simulink model "block_sensorless_startup_SMO_R2018a_sim_2020817"  (R2018a)
settings: Solver=ode1  StartTime=0.0  StopTime=1  FixedStep=1e-6  RelTol=1e-3  EnableMultiTasking=on
PreLoadFcn:
  | Psif= 0.003234246776455;  %magnet
  | Lq0 = 118e-6/2;  %inductance of q axis
  | Ld0 = 52.6e-6/2;   %inductance of d axis
  | R   =  43.73*0.5e-3;
  | 
  | Pn=4;       %poles pairs number
  | pi=3.1415926;
  | 
  | J=1.658254e-5*5;
  | Vdc=18;
undefined symbols (not defined in the file): DiscIntNeverNeededParam
libraries: powerlib x9, simulink x1
CloseFcn:
  | rtwprivate ssgencode ModelCloseRequest BLDC_baby_stroll_new_start
settings Model: DSRTSU_INTERNAL_RTI_VER=390  DSRTSU_INTERNAL_RTI_TYPE=rti1005  Creator=Engineer  LastModifiedBy=JinHua Luo
settings DataIOCC: LimitDataPoints=on  SaveFormat=Array  SignalLoggingSaveFormat=ModelDataLogs
settings OptimizationCC: BlockReduction=off  ConditionallyExecuteInputs=off  OptimizeBlockIOStorage=off  BufferReuse=off  GlobalBufferReuse=off  ExpressionFolding=off  EnableMemcpy=off  ExpressionDepthLimit=2147483647  LocalBlockOutputs=off  InitFltsAndDblsToZero=on  LifeSpan=inf  SimCompilerOptimization=on  OptimizeDataStoreBuffers=off  BusAssignmentInplaceUpdate=off
settings DebuggingCC: UnderspecifiedInitializationDetection=Classic  MergeDetectMultiDrivingBlocksExec=none  SolverPrmCheckMsg=warning  FcnCallInpInsideContextMsg=warning  StateNameClashWarn=warning  SFUnexpectedBacktrackingDiag=warning  SFNoUnconditionalDefaultTransitionDiag=warning  SFExecutionAtInitializationDiag=none
settings HardwareCC: ProdBitPerPointer=32  ProdBitPerSizeT=32  ProdBitPerPtrDiffT=32  ProdLargestAtomicFloat=None  ProdEndianess=BigEndian  ProdWordSize=32  ProdHWDeviceType=Generic->Custom  TargetIntDivRoundTo=Zero  TargetEndianess=BigEndian  TargetHWDeviceType=Generic->Custom
settings ModelReferenceCC: PropagateSignalLabelsOutOfModel=off
settings RTWCC: SystemTargetFile=rti1005.tlc  MakeCommand=make_rti  TemplateMakefile=rti1005.tmf  Description=dSPACE DS1005 Hardware Platform
settings CodeAppCC: StateflowObjectComments=on
settings STFCustomTargetCC: ParMdlRefBuildCompliant=on  GeneratePreprocessorConditionals=Disable all  CPPClassGenCompliant=on  SystemTargetFile=rti1005.tlc
settings GRTTargetCC: TargetLangStandard=C89/C90 (ANSI)  CompOptLevelCompliant=off  ConcurrentExecutionCompliant=off  GeneratePreprocessorConditionals=Disable all  CombineOutputUpdateFcns=off  MatFileLogging=off  GRTInterface=on  UseToolchainInfoCompliant=off  ExtModeMexFile=noextcomm
settings ConfigComp: CovMetricSettings=dw  CovHtmlReporting=on  CovSaveCumulativeToWorkspaceVar=on  CovSaveSingleToWorkspaceVar=on  CovExternalEMLEnable=off
settings SimscapeCC: SimscapeNormalizeSystem=off

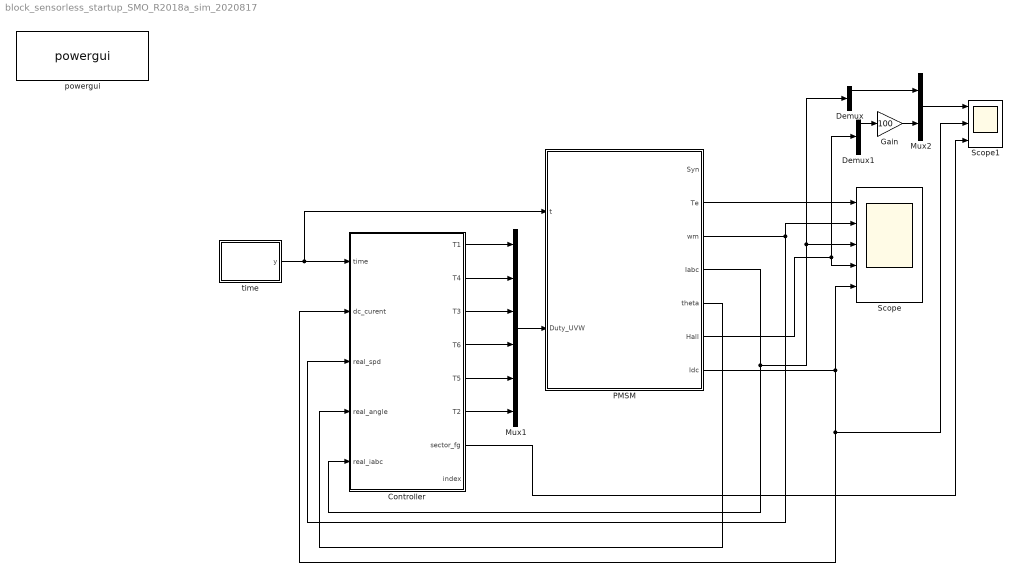
== system block_sensorless_startup_SMO_R2018a_sim_2020817 ==
  Controller : Subsystem
  Demux : Demux  Outputs=3
  Demux1 : Demux  Outputs=3
  Gain : Gain  Gain=100
  Mux1 : Mux  Inputs=6
  Mux2 : Mux  Inputs=2
  PMSM : Subsystem
  Scope : Scope  NumInputPorts=5
  Scope1 : Scope  NumInputPorts=3
  powergui : powerlib/powergui  Priority=2  SimulationMode=Discrete  SampleTime=1e-6  frequency=60  Iterations=50  frequencyindice=0  Pbase=100e6  ErrMax=1e-4  UnitsV=kV  UnitsW=MW  buscounter=0  FunctionMessages=off  echomessages=off  EnableUseOfTLC=off  CurrentSourceSwitches=off  DisableSnubberDevices=off  DisableRonSwitches=off  DisableVfSwitches=off  DisplayEquations=off  SolverType=Tustin/Backward Euler (TBE)  Interpol=off  ExternalGateDelay=off  methode=off  Ts=0  x0status=blocks  SPID=off  SwTol=0  HookPort=off  RestoreLinks=warning  ResistiveCurrentMeasurement=off  Frange=[0:2:500]  Ylog=off  Xlog=on  ShowGrid=off  save=off  variable=ZData  structure=0  ZoomFFT=on  StartTime=0.0  cycles=1  DisplayStyle=1  fundamental=60  FreqAxis=off  MaxFrequency=1000  frequencyindicesteady=1  RmsSteady=1  display=off
  time : MATLAB Function  TreatAsAtomicUnit=on
  wires:
  time/1(y) -> PMSM/1(t), Controller/1(time)
  Controller/1(T1) -> Mux1/1
  Controller/2(T4) -> Mux1/2
  Controller/3(T3) -> Mux1/3
  Controller/4(T6) -> Mux1/4
  Controller/5(T5) -> Mux1/5
  Controller/6(T2) -> Mux1/6
  Mux1/1 -> PMSM/2(Duty_UVW)
  PMSM/7(Idc) -> Scope/5, Controller/2(dc_curent), Scope1/2
  PMSM/2(Te) -> Scope/1
  PMSM/3(wm) -> Scope/2, Controller/3(real_spd)
  PMSM/4(Iabc) -> Controller/5(real_iabc), Demux/1, Scope/3
  PMSM/6(Hall) -> Demux1/1, Scope/4
  Demux/1 -> Mux2/1
  Demux1/1 -> Gain/1
  Mux2/1 -> Scope1/1
  Gain/1 -> Mux2/2
  Controller/7(sector_fg) -> Scope1/3
  PMSM/5(theta) -> Controller/4(real_angle)

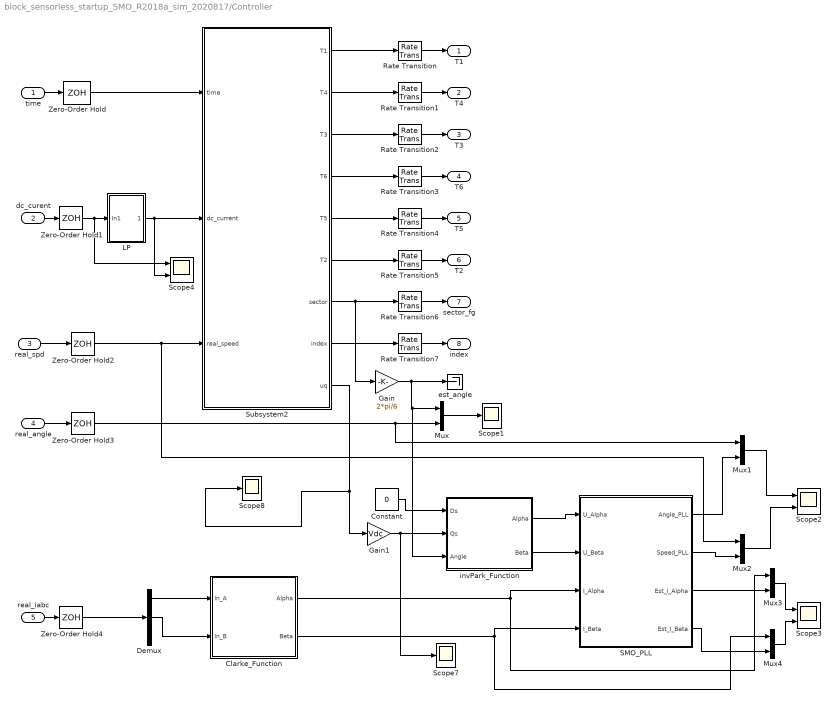
== system block_sensorless_startup_SMO_R2018a_sim_2020817/Controller ==
  time : Inport
  dc_curent : Inport  Port=2
  real_spd : Inport  Port=3
  real_angle : Inport  Port=4
  real_iabc : Inport  Port=5
  Clarke_Function : MATLAB Function  TreatAsAtomicUnit=on
  Constant : Constant  Value=0
  Demux : Demux  Outputs=3
  Gain : Gain  Gain=2*pi/6
  Gain1 : Gain  Gain=Vdc
  LP : Subsystem
  Mux{,1..4} (5 alike) : Mux  Inputs=2
  Rate Transition{,1..7} (8 alike) : RateTransition
  SMO_PLL : Subsystem
  Scope1 : Scope
  Scope2 : Scope  NumInputPorts=2
  Scope3 : Scope  NumInputPorts=2
  Scope4 : Scope  NumInputPorts=2
  Scope7 : Scope
  Scope8 : Scope
  Subsystem2 : Subsystem
  Zero-Order Hold{,1..4} (5 alike) : ZeroOrderHold  SampleTime=5e-5
  est_angle : Terminator
  invPark_Function : MATLAB Function  TreatAsAtomicUnit=on
  T1 : Outport
  T4 : Outport  Port=2
  T3 : Outport  Port=3
  T6 : Outport  Port=4
  T5 : Outport  Port=5
  T2 : Outport  Port=6
  sector_fg : Outport  Port=7
  index : Outport  Port=8
  wires:
  Subsystem2/1(T1) -> Rate Transition/1
  Subsystem2/2(T4) -> Rate Transition1/1
  Subsystem2/3(T3) -> Rate Transition2/1
  Subsystem2/4(T6) -> Rate Transition3/1
  Subsystem2/5(T5) -> Rate Transition4/1
  Subsystem2/6(T2) -> Rate Transition5/1
  time/1 -> Zero-Order Hold/1
  dc_curent/1 -> Zero-Order Hold1/1
  LP/1(Out1) -> Scope4/2, Subsystem2/2(dc_current)
  Zero-Order Hold/1 -> Subsystem2/1(time)
  Zero-Order Hold1/1 -> LP/1(In1), Scope4/1
  Rate Transition/1 -> T1/1
  Rate Transition1/1 -> T4/1
  Rate Transition2/1 -> T3/1
  Rate Transition3/1 -> T6/1
  Rate Transition4/1 -> T5/1
  Rate Transition5/1 -> T2/1
  Rate Transition6/1 -> sector_fg/1
  Rate Transition7/1 -> index/1
  Subsystem2/8(index) -> Rate Transition7/1
  real_spd/1 -> Zero-Order Hold2/1
  Zero-Order Hold2/1 -> Mux2/1, Subsystem2/3(real_speed)
  real_angle/1 -> Zero-Order Hold3/1
  real_iabc/1 -> Zero-Order Hold4/1
  Subsystem2/7(sector) -> Gain/1, Rate Transition6/1
  Gain/1 -> est_angle/1, invPark_Function/3(Angle), Mux/1
  Mux/1 -> Scope1/1
  Zero-Order Hold3/1 -> Mux1/1, Mux/2
  Demux/1 -> Clarke_Function/1(In_A)
  Demux/2 -> Clarke_Function/2(In_B)
  Clarke_Function/1(Alpha) -> SMO_PLL/3(I_Alpha), Mux3/1
  Clarke_Function/2(Beta) -> SMO_PLL/4(I_Beta), Mux4/1
  Subsystem2/9(uq) -> Scope8/1, Gain1/1
  invPark_Function/1(Alpha) -> SMO_PLL/1(U_Alpha)
  invPark_Function/2(Beta) -> SMO_PLL/2(U_Beta)
  Constant/1 -> invPark_Function/1(Ds)
  SMO_PLL/1(Angle_PLL) -> Mux1/2
  Mux1/1 -> Scope2/1
  SMO_PLL/2(Speed_PLL) -> Mux2/2
  Mux2/1 -> Scope2/2
  SMO_PLL/3(Est_I_Alpha) -> Mux3/2
  SMO_PLL/4(Est_I_Beta) -> Mux4/2
  Mux3/1 -> Scope3/1
  Mux4/1 -> Scope3/2
  Gain1/1 -> Scope7/1, invPark_Function/2(Qs)
  Zero-Order Hold4/1 -> Demux/1

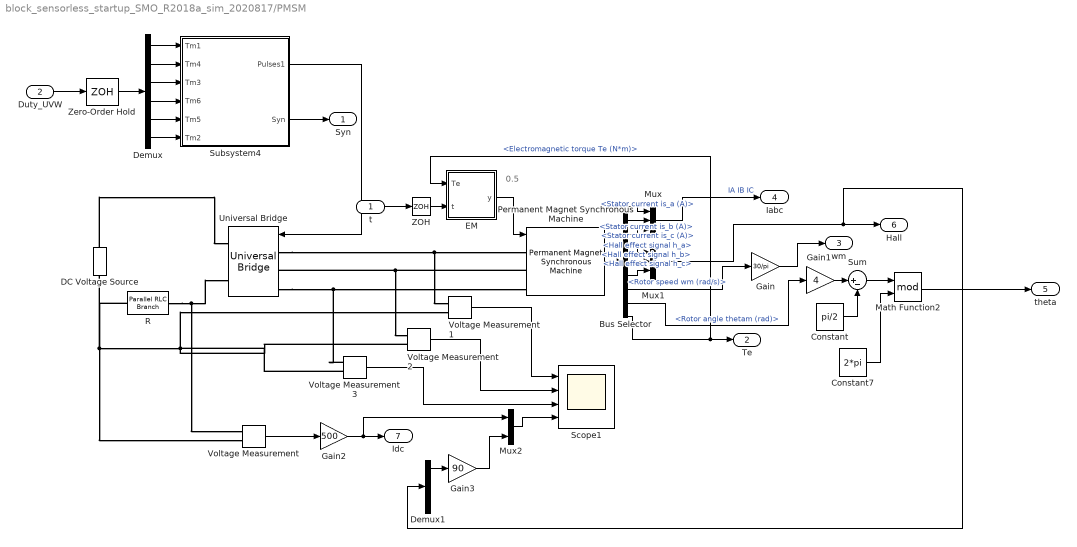
== system block_sensorless_startup_SMO_R2018a_sim_2020817/PMSM ==
  note: 0.5
  t : Inport
  Duty_UVW : Inport  Port=2  OutDataTypeStr=double
  Bus Selector : BusSelector  OutputSignals=Stator current is_a (A),Stator current is_b (A),Stator current is_c (A),Hall effect signal h_a,Hall effect signal h_b,Hall effect signal h_c,Rotor speed wm (rad/s),Rotor angle thetam (rad),Electromagnetic torque Te (N*m)
  Constant : Constant  Value=pi/2
  Constant7 : Constant  Value=2*pi
  DC Voltage Source : powerlib/Electrical Sources/DC Voltage Source  Amplitude=Vdc  Measurements=None
  Demux : Demux  Outputs=6
  Demux1 : Demux  Outputs=3
  EM : MATLAB Function  TreatAsAtomicUnit=on
  Gain : Gain  Gain=30/pi
  Gain1 : Gain  Gain=4
  Gain2 : Gain  Gain=500
  Gain3 : Gain  Gain=90
  Math Function2 : Math  Operator=mod  SaturateOnIntegerOverflow=on
  Mux : Mux  Inputs=3
  Mux1 : Mux  Inputs=3
  Mux2 : Mux  Inputs=2
  Permanent Magnet Synchronous Machine : powerlib/Machines/Permanent Magnet Synchronous Machine  NbPhases=3  FluxDistribution=Sinusoidal  RotorType=Salient-pole  MechanicalLoad=Torque Tm  PresetModel=No  ShowDetailedParameters=on  MeasurementBus=off  Resistance=R  Inductance=8.5e-3  dqInductances=[Ld0,Lq0]  La=0.000395  MachineConstant=Flux linkage established by magnets (V.s)  Flux=Psif  VoltageCst=2.3465  TorqueCst=0.019405  Flat=120  Mechanical=[J 100e-5 4]  PolePairs=4  InitialConditions=[0,0, 0,0]  InitialConditions5ph=[0 0 0 0 0 0]  TsPowergui=0  TsBlock=-1  RefAngle=90 degrees behind phase A axis (modified Park)
      settings: SourceProductName=Simscape Power Systems
  R : powerlib/Elements/Parallel RLC Branch  LConnTagsString=a  RConnTagsString=__new0  BranchType=R  Resistance=0.002  Inductance=1e-3  SetiL0=off  InitialCurrent=0  Capacitance=1e-6  Setx0=off  InitialVoltage=0  Measurements=None
  Scope1 : Scope  NumInputPorts=4
  Subsystem4 : Subsystem
  Sum : Sum  Inputs=|+-
  Universal Bridge : powerlib/Power Electronics/Universal Bridge  Arms=3  SnubberResistance=100  SnubberCapacitance=1e-5  Device=MOSFET / Diodes  Ron=3e-3  Lon=0  ForwardVoltages="[  0  0  ]"  ForwardVoltage=0  GTOparameters=[ 10e-6 , 20e-6 ]  IGBTparameters=[ 1e-6 , 2e-6 ]  Measurements=None  Measurements_2=None  converterType=Rectifier
  Voltage Measurement{,1..3} (4 alike) : powerlib/Measurements/Voltage Measurement  PhasorSimulation=off  OutputType=Complex  PSBequivalent=0
  ZOH : ZeroOrderHold  SampleTime=1e-6
  Zero-Order Hold : ZeroOrderHold  SampleTime=1e-6
  Syn : Outport
  Te : Outport  Port=2
  wm : Outport  Port=3
  Iabc : Outport  Port=4
  theta : Outport  Port=5
  Hall : Outport  Port=6
  Idc : Outport  Port=7
  wires:
  Permanent Magnet Synchronous Machine/1 -> Bus Selector/1
  Mux/1 -> Iabc/1  "IA IB IC"
  Bus Selector/7 -> Gain/1  "<Rotor speed wm (rad/s)>"
  Bus Selector/9 -> EM/1(Te), Te/1  "<Electromagnetic torque Te (N*m)>"
  Subsystem4/1(Pulses1) -> Universal Bridge/1
  Duty_UVW/1 -> Zero-Order Hold/1
  Subsystem4/2(Syn) -> Syn/1
  Constant/1 -> Sum/2
  Constant7/1 -> Math Function2/2
  Bus Selector/8 -> Gain1/1  "<Rotor angle thetam (rad)>"
  Math Function2/1 -> theta/1
  Gain/1 -> wm/1
  t/1 -> ZOH/1
  Demux/6 -> Subsystem4/6(Tm2)
  Demux/5 -> Subsystem4/5(Tm5)
  Demux/4 -> Subsystem4/4(Tm6)
  Demux/3 -> Subsystem4/3(Tm3)
  Demux/2 -> Subsystem4/2(Tm4)
  Demux/1 -> Subsystem4/1(Tm1)
  Zero-Order Hold/1 -> Demux/1
  ZOH/1 -> EM/2(t)
  Voltage Measurement/1 -> Gain2/1
  Gain2/1 -> Mux2/1, Idc/1
  EM/1(y) -> Permanent Magnet Synchronous Machine/1
  Mux1/1 -> Hall/1, Demux1/1
  Voltage Measurement1/1 -> Scope1/1
  Bus Selector/3 -> Mux/3  "<Stator current is_c (A)>"
  Bus Selector/2 -> Mux/2  "<Stator current is_b (A)>"
  Bus Selector/1 -> Mux/1  "<Stator current is_a (A)>"
  Bus Selector/5 -> Mux1/2  "<Hall effect signal h_b>"
  Bus Selector/6 -> Mux1/3  "<Hall effect signal h_c>"
  Bus Selector/4 -> Mux1/1  "<Hall effect signal h_a>"
  Voltage Measurement2/1 -> Scope1/2
  Voltage Measurement3/1 -> Scope1/3
  Demux1/1 -> Gain3/1
  Gain3/1 -> Mux2/2
  Mux2/1 -> Scope1/4
  Gain1/1 -> Sum/1
  Sum/1 -> Math Function2/1
  connections:
  Universal Bridge/LConn1 -- Permanent Magnet Synchronous Machine/LConn1 -- Voltage Measurement1/LConn1
  Permanent Magnet Synchronous Machine/LConn2 -- Universal Bridge/LConn2 -- Voltage Measurement2/LConn1
  Universal Bridge/LConn3 -- Voltage Measurement3/LConn1 -- Permanent Magnet Synchronous Machine/LConn3
  DC Voltage Source/RConn1 -- Universal Bridge/RConn1
  R/RConn1 -- Universal Bridge/RConn2 -- Voltage Measurement/LConn1
  R/LConn1 -- DC Voltage Source/LConn1 -- Voltage Measurement/LConn2 -- Voltage Measurement2/LConn2 -- Voltage Measurement3/LConn2 -- Voltage Measurement1/LConn2

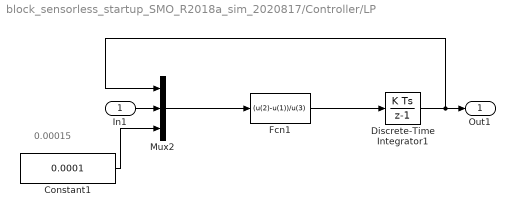
== system block_sensorless_startup_SMO_R2018a_sim_2020817/Controller/LP ==
  note: 0.00015
  In1 : Inport
  Constant1 : Constant  Value=0.0001  SampleTime=-1
  Discrete-Time Integrator1 : DiscreteIntegrator  SampleTime=-1  ICPrevOutput=DiscIntNeverNeededParam  ICPrevScaledInput=DiscIntNeverNeededParam
  Fcn1 : Fcn  Expr=(u(2)-u(1))/u(3)
  Mux2 : Mux  Inputs=3
  Out1 : Outport
  wires:
  Constant1/1 -> Mux2/3
  Mux2/1 -> Fcn1/1
  Fcn1/1 -> Discrete-Time Integrator1/1
  Discrete-Time Integrator1/1 -> Mux2/1, Out1/1
  In1/1 -> Mux2/2

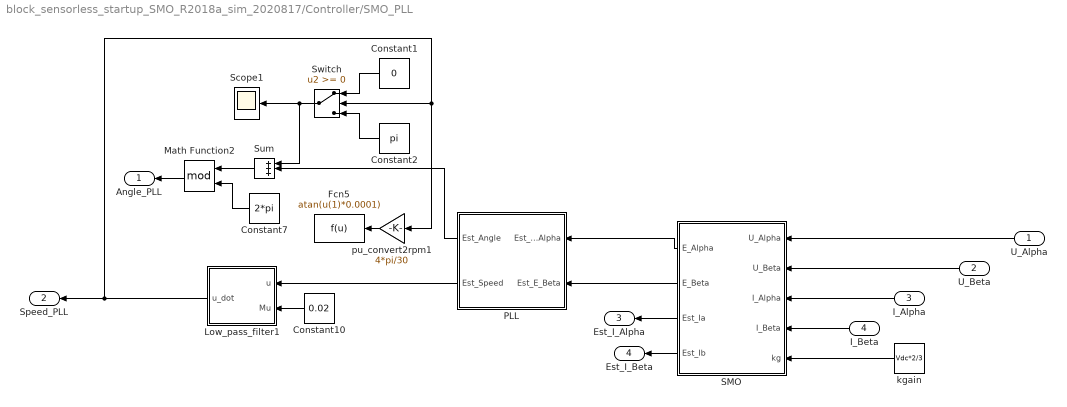
== system block_sensorless_startup_SMO_R2018a_sim_2020817/Controller/SMO_PLL ==
  U_Alpha : Inport
  U_Beta : Inport  Port=2
  I_Alpha : Inport  Port=3
  I_Beta : Inport  Port=4
  Constant1 : Constant  Value=0
  Constant10 : Constant  Value=0.02
  Constant2 : Constant  Value=pi
  Constant7 : Constant  Value=2*pi
  Fcn5 : Fcn  Expr=atan(u(1)*0.0001)
  Low_pass_filter1 : Subsystem
  Math Function2 : Math  Operator=mod  SaturateOnIntegerOverflow=on
  PLL : MATLAB Function  TreatAsAtomicUnit=on
  SMO : MATLAB Function  TreatAsAtomicUnit=on
  Scope1 : Scope
  Sum : Sum  Inputs=+++
  Switch : Switch
  kgain : Constant  Value=Vdc*2/3
  pu_convert2rpm1 : Gain  Gain=4*pi/30
  Angle_PLL : Outport
  Speed_PLL : Outport  Port=2
  Est_I_Alpha : Outport  Port=3
  Est_I_Beta : Outport  Port=4
  wires:
  Low_pass_filter1/1(u_dot) -> Speed_PLL/1, Switch/2, pu_convert2rpm1/1
  Constant10/1 -> Low_pass_filter1/2(Mu)
  I_Beta/1 -> SMO/4(I_Beta)
  I_Alpha/1 -> SMO/3(I_Alpha)
  U_Beta/1 -> SMO/2(U_Beta)
  U_Alpha/1 -> SMO/1(U_Alpha)
  Constant7/1 -> Math Function2/2
  PLL/2(Est_Speed) -> Low_pass_filter1/1(u)
  kgain/1 -> SMO/5(kg)
  Sum/1 -> Math Function2/1
  pu_convert2rpm1/1 -> Fcn5/1
  Math Function2/1 -> Angle_PLL/1
  SMO/1(E_Alpha) -> PLL/1(Est_E_Alpha)
  SMO/2(E_Beta) -> PLL/2(Est_E_Beta)
  PLL/1(Est_Angle) -> Sum/2
  Switch/1 -> Sum/1, Scope1/1
  SMO/4(Est_Ib) -> Est_I_Beta/1
  SMO/3(Est_Ia) -> Est_I_Alpha/1
  Constant2/1 -> Switch/3
  Constant1/1 -> Switch/1

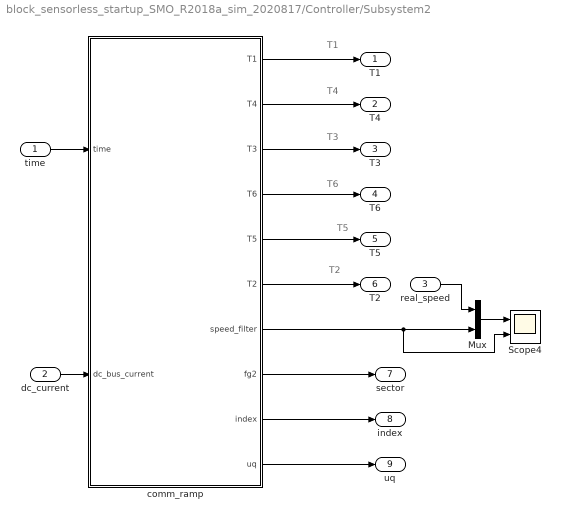
== system block_sensorless_startup_SMO_R2018a_sim_2020817/Controller/Subsystem2 ==
  note: T1
  note: T4
  note: T3
  note: T6
  note: T5
  note: T2
  time : Inport
  dc_current : Inport  Port=2
  real_speed : Inport  Port=3
  Mux : Mux  Inputs=2
  Scope4 : Scope  NumInputPorts=2
  comm_ramp : Subsystem  SystemSampleTime=4e-5
  T1 : Outport
  T4 : Outport  Port=2
  T3 : Outport  Port=3
  T6 : Outport  Port=4
  T5 : Outport  Port=5
  T2 : Outport  Port=6
  sector : Outport  Port=7
  index : Outport  Port=8
  uq : Outport  Port=9
  wires:
  time/1 -> comm_ramp/1(time)
  comm_ramp/1(T1) -> T1/1
  comm_ramp/2(T4) -> T4/1
  comm_ramp/3(T3) -> T3/1
  comm_ramp/4(T6) -> T6/1
  comm_ramp/6(T2) -> T2/1
  comm_ramp/5(T5) -> T5/1
  dc_current/1 -> comm_ramp/2(dc_bus_current)
  comm_ramp/9(index) -> index/1
  real_speed/1 -> Mux/1
  comm_ramp/7(speed_filter) -> Mux/2, Scope4/2
  Mux/1 -> Scope4/1
  comm_ramp/8(fg2) -> sector/1
  comm_ramp/10(uq) -> uq/1

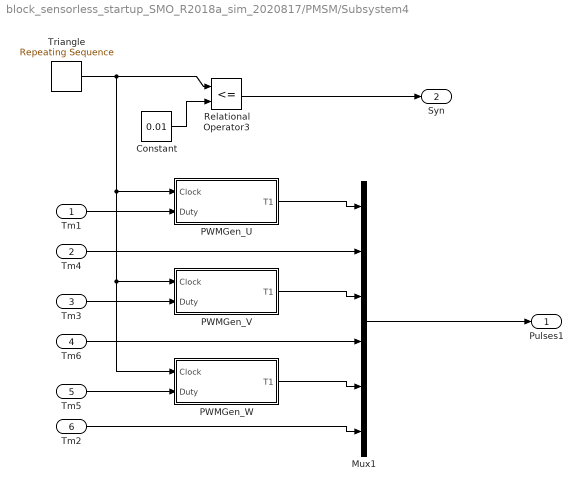
== system block_sensorless_startup_SMO_R2018a_sim_2020817/PMSM/Subsystem4 ==
  Tm1 : Inport
  Tm4 : Inport  Port=2
  Tm3 : Inport  Port=3
  Tm6 : Inport  Port=4
  Tm5 : Inport  Port=5
  Tm2 : Inport  Port=6
  Constant : Constant  Value=0.01
  Mux1 : Mux  Inputs=6
  PWMGen_U : Subsystem
  PWMGen_V : Subsystem
  PWMGen_W : Subsystem
  Relational Operator3 : RelationalOperator  Operator=<=  OutDataTypeStr=boolean  RndMeth=Nearest
  Triangle : simulink/Sources/Repeating Sequence  rep_seq_t=[0 0.000025 0.00005]  rep_seq_y=[0 1 0]
  Pulses1 : Outport
  Syn : Outport  Port=2
  wires:
  Mux1/1 -> Pulses1/1
  Tm1/1 -> PWMGen_U/2(Duty)
  Triangle/1 -> Relational Operator3/1, PWMGen_U/1(Clock), PWMGen_V/1(Clock), PWMGen_W/1(Clock)
  Relational Operator3/1 -> Syn/1
  Constant/1 -> Relational Operator3/2
  PWMGen_U/1(T1) -> Mux1/1
  Tm4/1 -> Mux1/2
  Tm2/1 -> Mux1/6
  Tm6/1 -> Mux1/4
  Tm3/1 -> PWMGen_V/2(Duty)
  Tm5/1 -> PWMGen_W/2(Duty)
  PWMGen_V/1(T1) -> Mux1/3
  PWMGen_W/1(T1) -> Mux1/5

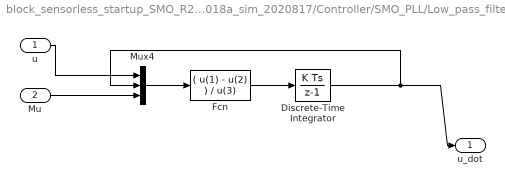
== system block_sensorless_startup_SMO_R2018a_sim_2020817/Controller/SMO_PLL/Low_pass_filter1 ==
  u : Inport
  Mu : Inport  Port=2
  Discrete-Time Integrator : DiscreteIntegrator  SampleTime=-1  RndMeth=Round  ICPrevOutput=DiscIntNeverNeededParam  ICPrevScaledInput=DiscIntNeverNeededParam
  Fcn : Fcn  Expr=( u(1) - u(2) ) / u(3)
  Mux4 : Mux  Inputs=3
  u_dot : Outport
  wires:
  Mu/1 -> Mux4/3
  u/1 -> Mux4/1
  Discrete-Time Integrator/1 -> u_dot/1, Mux4/2
  Fcn/1 -> Discrete-Time Integrator/1
  Mux4/1 -> Fcn/1

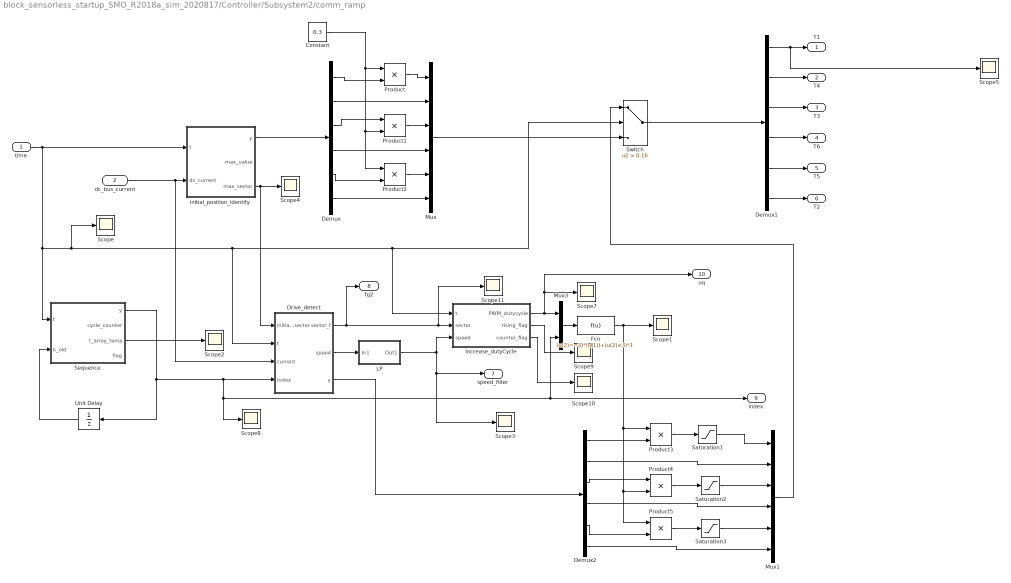
== system block_sensorless_startup_SMO_R2018a_sim_2020817/Controller/Subsystem2/comm_ramp ==
  time : Inport
  dc_bus_current : Inport  Port=2
  Constant : Constant  Value=0.3
  Demux : Demux  Outputs=6
  Demux1 : Demux  Outputs=6
  Demux2 : Demux  Outputs=6
  Drive_detect : MATLAB Function  TreatAsAtomicUnit=on
  Fcn : Fcn  Expr=(u(2)==3)*(u(1))+(u(2)<3)*1
  LP : Subsystem
  Mux : Mux  Inputs=6
  Mux1 : Mux  Inputs=6
  Mux3 : Mux  Inputs=2
  Product{,1..5} (6 alike) : Product  RndMeth=Zero
  Saturation1 : Saturate  UpperLimit=1  LowerLimit=0
  Saturation2 : Saturate  UpperLimit=1  LowerLimit=0
  Saturation3 : Saturate  UpperLimit=1  LowerLimit=0
  Scope{,1..5,7..11} (11 alike) : Scope
  Sequence : MATLAB Function  TreatAsAtomicUnit=on
  Switch : Switch  Criteria=u2 > Threshold  Threshold=0.16  OutDataTypeStr=double
  Unit Delay : UnitDelay  SampleTime=-1
  increase_dutyCycle : MATLAB Function  TreatAsAtomicUnit=on
  initial_position_identify : MATLAB Function  TreatAsAtomicUnit=on
  T1 : Outport
  T4 : Outport  Port=2
  T3 : Outport  Port=3
  T6 : Outport  Port=4
  T5 : Outport  Port=5
  T2 : Outport  Port=6
  speed_filter : Outport  Port=7
  fg2 : Outport  Port=8
  index : Outport  Port=9
  uq : Outport  Port=10
  wires:
  Demux/1 -> Product/2
  Demux/3 -> Product1/1
  Demux/5 -> Product2/2
  Constant/1 -> Product2/1, Product1/2, Product/1
  Demux1/1 -> Scope5/1, T1/1
  Demux1/2 -> T4/1
  Demux1/3 -> T3/1
  Demux1/4 -> T6/1
  Demux1/5 -> T5/1
  Demux1/6 -> T2/1
  Product/1 -> Mux/1
  Demux/2 -> Mux/2
  Product1/1 -> Mux/3
  Demux/4 -> Mux/4
  Product2/1 -> Mux/5
  Demux/6 -> Mux/6
  Mux/1 -> Switch/3
  Demux2/5 -> Product5/2
  dc_bus_current/1 -> Drive_detect/3(current), initial_position_identify/2(dc_current)
  initial_position_identify/1(y) -> Demux/1
  Demux2/3 -> Product4/1
  Product3/1 -> Saturation1/1
  Demux2/2 -> Mux1/2
  Product4/1 -> Saturation2/1
  Demux2/4 -> Mux1/4
  Product5/1 -> Saturation3/1
  Demux2/1 -> Product3/2
  Demux2/6 -> Mux1/6
  Drive_detect/3(y) -> Demux2/1
  initial_position_identify/3(max_sector) -> Drive_detect/1(initial_sector), Scope4/1
  Mux3/1 -> Fcn/1
  Saturation1/1 -> Mux1/1
  Saturation2/1 -> Mux1/3
  Saturation3/1 -> Mux1/5
  Mux1/1 -> Switch/1
  Fcn/1 -> Product3/1, Product5/1, Product4/2, Scope1/1
  Drive_detect/1(sector_f) -> increase_dutyCycle/2(sector), Scope11/1, fg2/1
  increase_dutyCycle/1(PWM_dutycycle) -> Mux3/1, Scope7/1, uq/1
  Drive_detect/2(speed) -> LP/1(In1)
  Sequence/1(y) -> Unit Delay/1, Drive_detect/4(index), Scope8/1, Mux3/2, index/1
  Unit Delay/1 -> Sequence/2(k_old)
  LP/1(Out1) -> increase_dutyCycle/3(speed), speed_filter/1, Scope3/1
  Switch/1 -> Demux1/1
  Sequence/3(t_array_temp) -> Scope2/1
  increase_dutyCycle/2(rising_flag) -> Scope9/1
  increase_dutyCycle/3(counter_flag) -> Scope10/1
  time/1 -> initial_position_identify/1(t), Scope/1, Drive_detect/2(t), Switch/2, increase_dutyCycle/1(t), Sequence/1(t)

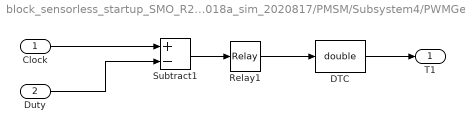
== system block_sensorless_startup_SMO_R2018a_sim_2020817/PMSM/Subsystem4/PWMGen_U ==
  Clock : Inport
  Duty : Inport  Port=2
  DTC : DataTypeConversion  OutDataTypeStr=double
  Relay1 : Relay  OnSwitchValue=0  OffSwitchValue=0  OnOutputValue=0  OffOutputValue=1
  Subtract1 : Sum  Inputs=+-
  T1 : Outport
  wires:
  Duty/1 -> Subtract1/2
  Clock/1 -> Subtract1/1
  DTC/1 -> T1/1
  Subtract1/1 -> Relay1/1
  Relay1/1 -> DTC/1

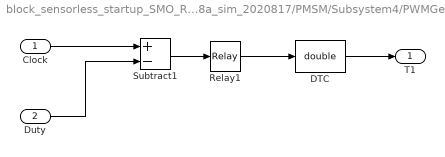
== system block_sensorless_startup_SMO_R2018a_sim_2020817/PMSM/Subsystem4/PWMGen_V ==
  Clock : Inport
  Duty : Inport  Port=2
  DTC : DataTypeConversion  OutDataTypeStr=double
  Relay1 : Relay  OnSwitchValue=0  OffSwitchValue=0  OnOutputValue=0  OffOutputValue=1
  Subtract1 : Sum  Inputs=+-
  T1 : Outport
  wires:
  Subtract1/1 -> Relay1/1
  DTC/1 -> T1/1
  Clock/1 -> Subtract1/1
  Duty/1 -> Subtract1/2
  Relay1/1 -> DTC/1

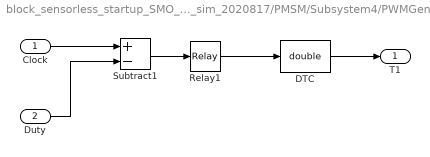
== system block_sensorless_startup_SMO_R2018a_sim_2020817/PMSM/Subsystem4/PWMGen_W ==
  Clock : Inport
  Duty : Inport  Port=2
  DTC : DataTypeConversion  OutDataTypeStr=double
  Relay1 : Relay  OnSwitchValue=0  OffSwitchValue=0  OnOutputValue=0  OffOutputValue=1
  Subtract1 : Sum  Inputs=+-
  T1 : Outport
  wires:
  Duty/1 -> Subtract1/2
  Clock/1 -> Subtract1/1
  DTC/1 -> T1/1
  Subtract1/1 -> Relay1/1
  Relay1/1 -> DTC/1

== system block_sensorless_startup_SMO_R2018a_sim_2020817/Controller/Subsystem2/comm_ramp/LP ==
  note: 0.00015
  In1 : Inport
  Constant1 : Constant  Value=0.001  SampleTime=-1
  Discrete-Time Integrator1 : DiscreteIntegrator  SampleTime=-1  ICPrevOutput=DiscIntNeverNeededParam  ICPrevScaledInput=DiscIntNeverNeededParam
  Fcn1 : Fcn  Expr=(u(2)-u(1))/u(3)
  Mux2 : Mux  Inputs=3
  Out1 : Outport
  wires:
  Constant1/1 -> Mux2/3
  Mux2/1 -> Fcn1/1
  Fcn1/1 -> Discrete-Time Integrator1/1
  Discrete-Time Integrator1/1 -> Mux2/1, Out1/1
  In1/1 -> Mux2/2

== matlab function block_sensorless_startup_SMO_R2018a_sim_2020817/time ==
  data: y output
function y = fcn()
%#eml

Ts=1e-6;

persistent t;

if isempty(t)
    t=0;
end

t=t+Ts;
y=t;

== matlab function block_sensorless_startup_SMO_R2018a_sim_2020817/Controller/Subsystem2/comm_ramp/initial_position_identify ==
  data: t input; y output; dc_current input; max_value output; max_sector output
function [y,max_value,max_sector] =fcn(t,dc_current)
%#eml
persistent  k dt dT  max_current sector dc_value dc_value_old s1_max s2_max s3_max s4_max s5_max s6_max max_array  flag1 flag2 flag3 flag4 flag5 flag6
 

if isempty(k)
    k=zeros(1,6);
end
if isempty(dt)
    dt=0.0005;  %0.0004s
end

if isempty(dT)
    dT=0.0006;  %0.00056s
end

if isempty(max_current)
    max_current=0;  
end

if isempty(sector)
    sector=0;  
end
if isempty(dc_value)
    dc_value=0;  
end
if isempty(dc_value_old)
    dc_value_old=0;  
end

if isempty(s1_max)
    s1_max=0;  
end
if isempty(s2_max)
    s2_max=0;  
end
if isempty(s3_max)
    s3_max=0;  
end
if isempty(s4_max)
    s4_max=0;  
end
if isempty(s5_max)
    s5_max=0;  
end
if isempty(s6_max)
    s6_max=0;  
end

if isempty(max_array)
    max_array=zeros(1,6);  
end

if isempty(flag1)
    flag1=0;  
end
if isempty(flag2)
    flag2=0;  
end
if isempty(flag3)
    flag3=0;  
end
if isempty(flag4)
    flag4=0;  
end
if isempty(flag5)
    flag5=0;  
end
if isempty(flag6)
    flag6=0;  
end





%%%%%%%%%%%%%%%%%%%%%%%%%%%%%%%%%%%%%%%%%%%%%%%%%%%%%%%%%%%%%%%%%%%%%%%%%%%%%%%%%%%

dc_value=dc_current;
if t<=0.1
  
    k=[0 0 0 0 0 0];
elseif (0.1<t && t<=(0.1+dt))                           %sector1  k=[1 0 0 1 0 1]  ; 
    k=[1 0 0 1 0 1]  ;  
    reset_counter=0;
elseif ((0.1+dt)<t && t<=(0.1+dt+dT)) 
                                
    k=[0 0 0 0 0 0]  ; 
      if (dc_value>dc_value_old)&& (flag1==0)
        s1_max=dc_value;
      else
          flag1=1;
          dc_value=0;
          dc_value_old=0;
     end
      max_array=[s1_max,0,0,0,0,0];
  
elseif ((0.1+dt+dT)<t && t<=(0.1+2*dt+dT) )            %sector4
    k=[0 1 1 0 1 0]  ;
  
     
elseif ((0.1+2*dt+dT)<t && t<=(0.1+2*dt+2*dT)) 
    
    k=[0 0 0 0 0 0]  ; 
    if (dc_value>dc_value_old)&& (flag4==0)
        s4_max=dc_value;
    else
         flag4=1;
         dc_value=0;
         dc_value_old=0;
    end
    max_array=[s1_max,0,0,s4_max,0,0];
   
elseif ((0.1+2*dt+2*dT)<t && t<=(0.1+3*dt+2*dT))         %sector2
    k=[1 0 1 0 0 1] ;
    %  k=[0 0 0 0 0 0]  ;
elseif ((0.1+3*dt+2*dT)<t && t<=(0.1+3*dt+3*dT)) 
   
   k=[0 0 0 0 0 0]  ; 
     if (dc_value>dc_value_old)&& (flag2==0)
        s2_max=dc_value;
     else
         flag2=1;
         dc_value=0;
         dc_value_old=0;
     end
     max_array=[s1_max,s2_max,0,s4_max,0,0];
    
elseif ((0.1+3*dt+3*dT)<t && t<=(0.1+4*dt+3*dT))         %sector5
    k=[0 1 0 1 1 0] ;
   
elseif ((0.1+4*dt+3*dT)<t && t<=(0.1+4*dt+4*dT)) 
   
   k=[0 0 0 0 0 0]  ; 
      if (dc_value>dc_value_old)&& (flag5==0)
        s5_max=dc_value;
      else
          flag5=1;
          dc_value=0;
          dc_value_old=0;
     end
     max_array=[s1_max,s2_max,0,s4_max,s5_max,0];
    
elseif ((0.1+4*dt+4*dT)<t && t<=(0.1+5*dt+4*dT))           %sector3
    k=[0 1 1 0 0 1]; 
     
     
elseif ((0.1+5*dt+4*dT)<t && t<=(0.1+5*dt+5*dT)) 
   
  k=[0 0 0 0 0 0]  ; 
    if (dc_value>dc_value_old)&& (flag3==0)
        s3_max=dc_value;
    else
      flag3=1;
      dc_value=0;
      dc_value_old=0;
    end
     max_array=[s1_max,s2_max,s3_max,s4_max,s5_max,0];
     
    
elseif ((0.1+5*dt+5*dT)<t && t<=(0.1+6*dt+5*dT))          %sector6
    k=[1 0 0 1 1 0];
    
elseif t>(0.1+6*dt+5*dT)&& t<(0.1+7*dt+5*dT)
  
    k=[0 0 0 0 0 0]  ; 
    if (dc_value>dc_value_old)&& (flag6==0)
        s6_max=dc_value;
    else
       flag6=1;
       dc_value=0;
       dc_value_old=0;
    end
     max_array=[s1_max,s2_max,s3_max,s4_max,s5_max,s6_max];
    [max_current,sector]=max(max_array);
elseif t>(0.1+7*dt+5*dT)&& t<(0.1+7*dt+5*dT+0.05)
     k=[0 0 0 0 0 0];
     flag1=0;
     flag2=0;
     flag3=0;
     flag4=0;
     flag5=0;
     flag6=0;
     dc_value=0;
     dc_value_old=0;
    
end


dc_value_old=dc_value;

y=k;
max_value=dc_value;%max_current;
max_sector=sector;

== matlab function block_sensorless_startup_SMO_R2018a_sim_2020817/PMSM/EM ==
  data: Te input; t input; y output
function y = fcn(Te,t)
%#eml

if t<0.165
    y=Te;
else
    y=0.25;
end

== matlab function block_sensorless_startup_SMO_R2018a_sim_2020817/Controller/Subsystem2/comm_ramp/increase_dutyCycle ==
  data: t input; sector input; PWM_dutycycle output; speed input; rising_flag output; counter_flag output
function [PWM_dutycycle,rising_flag,counter_flag]  = fcn(t,sector,speed)
%#codegen

Ts=5e-5;
persistent sector_rising_edge sector_old counter dutycycle stall_flag

if isempty(sector_rising_edge)
    sector_rising_edge=0;
end

if isempty(sector_old)
    sector_old=0;
end

if isempty(dutycycle)
    dutycycle=0.12;   %  dutycycle=0.18 for 20V DC bus voltage
end

if isempty(counter)
    counter=0;
end

if isempty(stall_flag)
    stall_flag=0;
end


%%%%%%%%%%%%%%%%%%%%%%%%%%%%%%%%%%%%%%%%%%%%%%
if t<0.16
    dutycycle=0.12;  %0.18
elseif t>0.16
    
        if (sector> sector_old)||((sector< sector_old)&&(sector_old==6))
            sector_rising_edge=1;
        else
            sector_rising_edge=0;
        end

        if (sector==sector_old)%&&(counter>=0.08/4e-5)
            counter=counter+1;
            if counter>= (0.15/Ts)  %if counter>= (0.05/4e-5)
                stall_flag=1;
            end
        else
            counter=0;
            stall_flag=0;


        end
        if ((speed<350)&&(sector_rising_edge==1))||(stall_flag==1)
            dutycycle=dutycycle+0.005;%0.01
                if dutycycle>=0.3   % 0.55
                    dutycycle=0.3;  % 0.55
                    stall_flag=0;
                end        
        end
end


sector_old=sector;
%%%%%%%%%%%%%%%%%%%%%%%%%%%%%%%%%%%%%%%%%%%%%%%%%%%%%%%%%%%%%%%%%%%%

PWM_dutycycle=dutycycle;
rising_flag=stall_flag;
counter_flag=counter;

== matlab function block_sensorless_startup_SMO_R2018a_sim_2020817/Controller/Subsystem2/comm_ramp/Sequence ==
  data: t input; y output; cycle_counter output; t_array_temp output; k_old input; flag output
function [y,cycle_counter,t_array_temp,flag] = fcn(t,k_old)
%#eml

Ts=5e-5;
persistent sector k t_array t_drive_diode t0 t1  t2 t_detect_diode counter one_cycle_counter over_flag

if isempty(sector)
    sector=3;
end

if isempty(k)
    k=0;
end

if isempty(t_array)
    %t_array=[0.030 0.018 0.016 0.014 0.012 0.010 0.008 0.006 0.004 0.003]; 
    t_array=0.01;% initial pulse width 0.01s,10ms
end

if isempty(t_drive_diode)
    t_drive_diode=0.0005*0.8;%0.5ms  drive doide freewheeling
end
if isempty(t0)
    t0=0.00005*0;% 0ms, mosfet channels are all set to 0
end
if isempty(t1)
    t1=0.0002;%0.5ms t1 detect time
end

if isempty(t2)
    t2=0.0002;%0.5ms t1 detect time
end

if isempty(t_detect_diode)
    t_detect_diode=0.0002;%0.5ms  detect diode freewheeling time
end

if isempty(counter)
    counter=0;
end

if isempty(one_cycle_counter)
    one_cycle_counter=0;
end

if isempty(over_flag)
    over_flag=0;
end


%%%%%%%%%%%%%%%%%%%%%%%%%%%%%%%%%%%%%%%%%%%%%%%%
if t<=0.16
    k=0;
elseif t>0.16
            if sector==3
                k=3;
                 if k_old<k
                     one_cycle_counter=one_cycle_counter+1;
                     if one_cycle_counter>=1
                         t_array=t_array-0.001;  %0.0004;
                         if t_array<=0.005   %0.003 for 600rpm,0.003
                             t_array=0.005;  %0.003
                             over_flag=5;
                         end
                         one_cycle_counter=0;
                     end
                 end    
                counter=counter+1;
                if counter>=(t_array/Ts)
                    sector=0.8;
                    counter=0;
                end
            elseif sector==0.8
                k=0.8;
                counter=counter+1;
                if counter>=(t_drive_diode/Ts)
                    sector=1.4;  %1.2
                    counter=0;
                end
%             elseif sector==1.2
%                 k=1.2;
%                 counter=counter+1;
%                 if counter>=(t0/Ts)
%                     sector=1.4;
%                     counter=0;
%                 end
            elseif sector==1.4
                k=1.4;
                counter=counter+1;
                if counter>=(t1/Ts)
                    sector=1.8;
                    counter=0;
                end
            elseif sector==1.8
                k=1.8;
                counter=counter+1;
                if counter>=(t_detect_diode/Ts)
                    sector=2.5; %2.1
                    counter=0;
                end
%             elseif sector==2.1
%                 k=2.1;
%                 counter=counter+1;
%                 if counter>=(t0/Ts)
%                     sector=2.5;
%                     counter=0;
%                 end
            elseif sector==2.5
                k=2.5;
                counter=counter+1;
                if counter>=(t2/Ts)
                    sector=2.6;
                    counter=0;
                end
            elseif sector==2.6
                k=2.6;
                counter=counter+1;
                if counter>=(t_detect_diode/Ts)
                    sector=3;  %2.8
                    counter=0;
                end
%             elseif sector==2.8
%                 k=2.8;
%                  counter=counter+1;
%                 if counter>=(t0/Ts)
%                     sector=3;
%                     counter=0;
%                 end
            end
           
end


y = k;
cycle_counter=one_cycle_counter;
t_array_temp=t_array;
% cycle_counter=k;
% t_array_temp=k_old;
flag=over_flag;

== matlab function block_sensorless_startup_SMO_R2018a_sim_2020817/Controller/Subsystem2/comm_ramp/Drive_detect ==
  data: initial_sector input; sector_f output; speed output; t input; current input; y output; index input
function [sector_f,speed,y] =fcn(initial_sector,t,current,index)
%#eml
persistent  k dc_value dc_value_old s11_max s12_max s21_max s22_max s31_max s32_max s41_max s42_max s51_max s52_max s61_max s62_max 
persistent sector counter1 counter2 counter3 counter4 counter5 counter6 counter1_temp counter2_temp counter3_temp counter4_temp counter5_temp counter6_temp speed_counter  speed_judge
persistent   index1_temp  bEMF_flag    

if isempty(k)
    k=[0 0 0 0 0 0];
end

if isempty(dc_value)
    dc_value=0;
end

if isempty(dc_value_old)
    dc_value_old=0;
end


if isempty(s11_max)
    s11_max=0;
end

if isempty(s12_max)
    s12_max=0;
end

if isempty(s21_max)
    s21_max=0;
end

if isempty(s22_max)
    s22_max=0;
end
if isempty(s31_max)
    s31_max=0;
end

if isempty(s32_max)
    s32_max=0;
end
if isempty(s41_max)
    s41_max=0;
end

if isempty(s42_max)
    s42_max=0;
end
if isempty(s51_max)
    s51_max=0;
end

if isempty(s52_max)
    s52_max=0;
end
if isempty(s61_max)
    s61_max=0;
end

if isempty(s62_max)
    s62_max=0;
end

if isempty(sector)
    sector=1;
end

if isempty(counter1)
    counter1=0;
end

if isempty(counter2)
    counter2=0;
end

if isempty(counter3)
    counter3=0;
end

if isempty(counter4)
    counter4=0;
end
if isempty(counter5)
    counter5=0;
end

if isempty(counter6)
    counter6=0;
end

if isempty(counter1_temp)
    counter1_temp=5000;
end

if isempty(counter2_temp)
    counter2_temp=5000;
end

if isempty(counter3_temp)
    counter3_temp=5000;
end

if isempty(counter4_temp)
    counter4_temp=5000;
end
if isempty(counter5_temp)
    counter5_temp=5000;
end

if isempty(counter6_temp)
    counter6_temp=5000;
end

if isempty(speed_counter)
    speed_counter=5000;
end



if isempty(speed_judge)
    speed_judge=0;
end

if isempty(index1_temp)
    index1_temp=0;
end

if isempty(bEMF_flag)
    bEMF_flag=0;
end







%%%%%%%%%%%%%%%%%%%%%%%%%%%%%%%%%%%%%%%%%%%%%%%%%%%%%%%%%%%%



dc_value=current;

%%%%%%%    
if t<=0.16  
    k=[0 0 0 0 0 0];
     sector=initial_sector;  
elseif t>0.16   
   if sector==1
 %%%%%%%%%%%%%%%%%%%%%%%%%%%%%%%%%%%%%%%%%%%%%%%%%%%%%%%%%   
       %%%%%%%%%%%%%%%%%%%%%%%%%%% 
            counter1=counter1+1;
            counter6_temp=counter6;
            counter5=0;
      %%%%%%%%%%%%%%%%%%%%%%%%%%%%%%%%%%%%%
            if (index==3) %  B+C-drive. 
               %k=[0 0 0 1 1 0]; 
               k=[0 0 1 0 0 1]; 
                s61_max=0;
                s62_max=0;
            elseif (index==0.8)
                  k=[0 0 0 0 0 1]*0;      % diode freewheeling     
%                 k=[0 0 0 1 0 1];      % diode freewheeling   
                          
            elseif (index==1.4) %  first inject A+B-C- detect,
                k=[0.15 0 0 1 0 1];  % k=[0.15 0 0 1 0 1];
                
            elseif (index==1.8)
                  k=[0 0 0 1 0 1]*0;
%                 k=[0 1 0 1 0 1];

                 if (dc_value>=dc_value_old)
                    s11_max=dc_value;
                 else
                  dc_value=0;
                  dc_value_old=0;
                 end
                                                
            elseif (index==2.5) %inject A+B+C- detect.
                 k=[0.15 0 0.15 0 0 1];
                 
            elseif (index==2.6)
                  k=[0 0 0 0 0 1];
%                 k=[0 1 0 1 0 1];

                  if (dc_value>=dc_value_old)
                            s12_max=dc_value;
                  else
                          dc_value=0;
                          dc_value_old=0;
                  end
                  
              %    if (abs(s11_max-s12_max)<=0.15)&&(s11_max>0.5)      %  if (s11_max<s12_max)&&(s11_max>0.5)
                 if (s11_max<s12_max)&&(s11_max>0.5)
                       sector=2;
                  end  
             
            end
            
    
   elseif sector==2    
                                          
   %%%%%%%%%%%%%%%%%%%%%%%%%%%%%%%%%%%%%%%%%%%%%%%%%%%%%%%%%%%%%%%%%%%%%%%%%%%%%%%%%%   
             index1_temp=0; 
             counter2=counter2+1;
             counter1_temp=counter1;
             counter6=0;
          %%%%%%%%%%%%%%%%%%%%%%%%%%%%%%%%%%%%%   
                if (index==3) %  %%% B+A- drive
                 %  k=[1 0 0 1 0 0];   
                    k=[0 1 1 0 0 0]; 
                    s11_max=0;
                    s12_max=0;
                elseif (index==0.8)
                     k=[0 1 0 0 0 0]*0;      % diode freewheeling  
%                    k=[0 1 0 1 0 0];        

                elseif (index==1.4) %  first inject A+B+C- detect,
                    k=[0.15 0 0.15 0 0 1];  % k=[0.15 0 0.15 0 0 1]; 
          
                elseif (index==1.8)      % diode freewheeling    
                      k=[0 0 0 0 0 1]*0;  
%                     k=[0 1 0 1 0 1];  

                     if (dc_value>=dc_value_old)
                        s21_max=dc_value;
                     else
                      dc_value=0;
                      dc_value_old=0;
                     end
                                

                elseif (index==2.5) %inject A-B+C- drive motor.
                     k=[0 1 0.15 0 0 1];

                elseif (index==2.6)
                     k=[0 1 0 0 0 1]*0;
%                     k=[0 1 0 1 0 1];

                      if (dc_value>=dc_value_old)
                                s22_max=dc_value;
                      else
                              dc_value=0;
                              dc_value_old=0;
                      end
                      
                  %    if (abs(s21_max-s22_max)<=0.15)&&(s21_max>0.5)  % if (s21_max<s22_max)&&(s21_max>0.5)
                     if (s21_max<s22_max)&&(s21_max>0.5)
                           sector=3;
                      end  
                      
                end          
                                        
        
    elseif sector==3
       
 %%%%%%%%%%%%%%%%%%%%%%%%%%%%%%%%%%%%%%%%%%%%%%%%%%%%%%%%%%%%%%%%%%%%%     
          counter3=counter3+1;
          counter2_temp=counter2;
          counter1=0;
          %%%%%%%%%%%%%%%%%%%%%%%%%%%%%%%%%%%%%%%
                if (index==3) %  C+A- drive
                 %  k=[1 0 0 0 0 1]; 
                   k=[0 1 0 0 1 0];    
                    s21_max=0;
                    s22_max=0;
                elseif (index==0.8)
                   k=[0 0 0 0 0 0];      % diode freewheeling   
%                    k=[0 1 0 0 0 1]; 
                elseif (index==1.4) % first inject A-B+C- detect,
                    k=[0 1 0.15 0 0 1];  % k=[0 1 0.15 0 0 1]; 
          
                elseif (index==1.8)      % diode freewheeling   
                      k=[0 1 0 0 0 1]*0;  
%                     k=[0 1 0 1 0 1];  

                     if (dc_value>=dc_value_old)
                        s31_max=dc_value;
                     else
                      dc_value=0;
                      dc_value_old=0;
                     end
                               

                elseif (index==2.5) %inject A-B+C+ drive motor.
                     k=[0 1 0.15 0 0.15 0];
                elseif (index==2.6)
                      k=[0 1 0 0 0 0]*0;
%                     k=[0 1 0 1 0 1];

                      if (dc_value>=dc_value_old)
                                s32_max=dc_value;
                      else
                              dc_value=0;
                              dc_value_old=0;
                      end

                 %     if (abs(s31_max-s32_max)<=0.15)&&(s31_max>0.5)    % if (s31_max<s32_max)&&(s31_max>0.5)
                     if (s31_max<s32_max)&&(s31_max>0.5)
                           sector=4;
                      end  
                      
                end 
                    
    elseif sector==4
         
  %%%%%%%%%%%%%%%%%%%%%%%%%%%%%%%%%%%%%%%%%%%%%%%%%%%%%%%%%%%%% 
           counter4=counter4+1;
           counter3_temp=counter3;
           counter2=0;
           %%%%%%%%%%%%%%%%%%%%%%%%%%%%%%%%%%%
                 if (index==3) %% C+B- drive
                 %  k=[0 0 1 0 0 1];   
                    k=[0 0 0 1 1 0];    
                    s31_max=0;
                    s32_max=0;
                elseif (index==0.8)
                       k=[0 0 0 1 0 0]*0;      % diode freewheeling  
%                      k=[0 0 0 1 0 1];  

                elseif (index==1.4) %first inject A-B+C+ detect,
                    k=[0 1 0.15 0 0.15 0];  % k=[0 1 0.15 0 0.15 0]; 
          
                elseif (index==1.8)      % diode freewheeling   
                      k=[0 1 0 0 0 0]*0;  
%                     k=[0 1 0 1 0 1];  

                     if (dc_value>=dc_value_old)
                        s41_max=dc_value;
                     else
                      dc_value=0;
                      dc_value_old=0;
                     end
                               
                elseif (index==2.5) %inject A-B-C+ drive motor.
                     k=[0 1 0 1 0.15 0];
                % k=[0 1 0 1 0.15 0];

                elseif (index==2.6)
                      k=[0 1 0 1 0 0]*0;
%                     k=[0 1 0 1 0 1];

                      if (dc_value>=dc_value_old)
                                s42_max=dc_value;
                      else
                              dc_value=0;
                              dc_value_old=0;
                      end

                 %     if (abs(s41_max-s42_max)<=0.15)&&(s41_max>0.5)  % if (s41_max<s42_max)&&(s41_max>0.5)
                     if (s41_max<s42_max)&&(s41_max>0.5)
                           sector=5;
                      end  
                        
                 end
                
               
                    
    elseif sector==5
        
  %%%%%%%%%%%%%%%%%%%%%%%%%%%%%%%%%%%%%%%%%%%%%%%%%%%%%%%%%    
           counter5=counter5+1;
           counter4_temp=counter4;
           counter3=0;
         %%%%%%%%%%%%%%%%%%%%%%%%%%%%%%%%%
                if (index==3) %  A+B- drive
                  % k=[0 1 1 0 0 0];  
                    k=[1 0 0 1 0 0];    
                    s41_max=0;
                    s42_max=0;
                elseif (index==0.8)
                       k=[0 0 0 1 0 0]*0;      % diode freewheeling     
%                      k=[0 1 0 1 0 0];  

                elseif (index==1.4) % first inject A-B-C+ detect,
                    k=[0 1 0 1 0.15 0];  %  k=[0 1 0 1 0.15 0]; 
          
                elseif (index==1.8)      % diode freewheeling    
                    k=[0 1 0 1 0 0]*0; 
%                     k=[0 1 0 1 0 1];  

                     if (dc_value>=dc_value_old)
                        s51_max=dc_value;
                     else
                      dc_value=0;
                      dc_value_old=0;
                     end

                elseif (index==2.5) %inject A+B-C+ drive motor.
                     k=[0.15 0 0 1 0.15 0];

                elseif (index==2.6)
                      k=[0 0 0 1 0 0]*0;
%                     k=[0 1 0 1 0 1];

                      if (dc_value>=dc_value_old)
                                s52_max=dc_value;
                      else
                              dc_value=0;
                              dc_value_old=0;
                      end

                  %    if (abs(s51_max-s52_max)<=0.15)&&(s51_max>0.5)  %if (s51_max<s52_max)&&(s51_max>0.5)
                      if (s51_max<s52_max)&&(s51_max>0.5)
                           sector=6;
                      end  
                     
   
                 end
                   
    elseif sector==6       
 %%%%%%%%%%%%%%%%%%%%%%%%%%%%%%%%%%%%%%%%%%%%%%%%%%%%%%%%%%%%%%%%%%%%%%%       
     counter6=counter6+1;
     counter5_temp=counter5;
           counter4=0;
           %%%%%%%%%%%%%%%%%%%%%%%
                 if (index==3) % A+C- drive
                 %  k=[0 1 0 0 1 0];   
                    k=[1 0 0 0 0 1];  
                    s51_max=0;
                    s52_max=0;
                elseif (index==0.8)
                      k=[0 0 0 0 0 1]*0;      % diode freewheeling     
%                     k=[0 1 0 0 0 1];  

                elseif (index==1.4) % first inject A+B-C+ detect,
                    k=[0.15 0 0 1 0.15 0];  % k=[0.15 0 0 1 0.15 0]; 
                    
                elseif (index==1.8)      % diode freewheeling   
                     k=[0 0 0 1 0 0]*0; 
%                     k=[0 1 0 1 0 1];  

                     if (dc_value>=dc_value_old)
                        s61_max=dc_value;
                     else
                      dc_value=0;
                      dc_value_old=0;
                     end
                               

                elseif (index==2.5) %inject A+B-C- drive motor.
                     k=[0.15 0 0 1 0 1];

                elseif (index==2.6)
                      k=[0 0 0 1 0 1]*0;
%                     k=[0 1 0 1 0 1];
 
                      if (dc_value>=dc_value_old)
                                s62_max=dc_value;
                      else
                              dc_value=0;
                              dc_value_old=0;
                      end

                   %   if (abs(s61_max-s62_max)<=0.15)&&(s61_max>0.5)   % if (s61_max<s62_max)&&(s61_max>0.5)
                      if (s61_max<s62_max)&&(s61_max>0.5)
                           sector=1;
                      end  
                     
                 end
                      
   end
  
    speed_counter=(counter1_temp+counter2_temp+counter3_temp+counter4_temp+counter5_temp+counter6_temp)/6;
    speed_judge=60/(speed_counter*6*5e-5*4);  % pole-pairs is 4,
   
end

dc_value_old=dc_value;

%%%%%%%%%%%%%%%%%%%%%%%%%%%%%%%%%%%%%%%%%%%%%%%%%%%%


sector_f=sector;
speed=speed_judge;
y=k;

== matlab function block_sensorless_startup_SMO_R2018a_sim_2020817/Controller/invPark_Function ==
  data: Alpha output; Ds input; Beta output; Qs input; Angle input
function [Alpha,Beta] = fcn(Ds,Qs,Angle)
%#eml

persistent  Sine  Cosine 

if isempty(Sine)
    Sine  = 0;
end

if isempty(Cosine)
    Cosine  = 0;
end

Sine   = sin(Angle);
Cosine = cos(Angle);


Alpha = Ds * Cosine - Qs  * Sine;
Beta  = Qs * Cosine + Ds  * Sine;

== matlab function block_sensorless_startup_SMO_R2018a_sim_2020817/Controller/Clarke_Function ==
  data: In_A input; In_B input; Alpha output; Beta output
function [Alpha,Beta] = fcn(In_A,In_B)
%#eml

Alpha = In_A;

Beta  = 0.57735026918963 * (2*In_B + In_A);

== matlab function block_sensorless_startup_SMO_R2018a_sim_2020817/Controller/SMO_PLL/PLL ==
  data: Est_E_Alpha input; Est_Angle output; Est_E_Beta input; Est_Speed output
function [Est_Angle,Est_Speed] = fcn(Est_E_Alpha,Est_E_Beta)
%#eml

wb = 4 * 2 *pi/60;
T  = 5e-5;
F = wb * T;

K1 = 200^2;
K2 =1/200;


persistent  Error_Angle     
persistent  SpdMax  SpdMin
persistent  Up      Ui  
persistent  SpdSat  SpdPreSat  
persistent  Angle
persistent  PreSpd     Spd


if isempty(Error_Angle)
    Error_Angle  = 0;
end

if isempty(SpdMax)
    SpdMax  = 6000;
end

if isempty(SpdMin)
    SpdMin  = -6000;
end


if isempty(Up)
    Up = 0;
end

if isempty(Ui)
    Ui = 0;
end

if isempty(SpdPreSat)
    SpdPreSat = 0;
end

if isempty(SpdSat)
    SpdSat = 0;
end

if isempty(Angle)
    Angle = 0;
end

if isempty(Spd)
    Spd = 0;
end

if isempty(PreSpd)
    PreSpd = 0;
end


Error_Angle  = -Est_E_Alpha * cos(Angle) -Est_E_Beta * sin(Angle);

Up = K2 * Error_Angle ;

Ui = Ui + T * Error_Angle;
if (Ui > SpdMax)
    Ui = SpdMax;
elseif((Ui < SpdMin))
    Ui = SpdMin;
end
    

SpdPreSat =  K1*(Up + Ui);

Spd = 0.1*(SpdPreSat - PreSpd) + PreSpd;


Angle = mod((Angle + SpdPreSat * F),(2*pi)) ;


PreSpd = Spd;

Est_Angle = Angle; 
Est_Speed = Spd;

== matlab function block_sensorless_startup_SMO_R2018a_sim_2020817/Controller/SMO_PLL/SMO ==
  data: U_Alpha input; E_Alpha output; U_Beta input; I_Alpha input; I_Beta input; E_Beta output; Est_Ia output; Est_Ib output; kg input
function [E_Alpha,E_Beta,Est_Ia,Est_Ib] = fcn(U_Alpha,U_Beta,I_Alpha,I_Beta,kg)
%#eml

persistent  Est_I 
persistent  Pre_U 
persistent  Est_E
persistent  Error_I
persistent  Z


L  = 90e-6/2;
R  =  43.73e-3/2;
T  = 5e-5;
Kslide = kg;     %SMO gain  Kslide = 10
Kslf   = 0.5;    % 0.5 parameter for low-pass filter 

Error =0.5;  %  0.5 bounary width(A)

F = 1-R*T/L;

G = T/L;


%Estimated Current
if isempty(Est_I)
    Est_I = struct('Alpha',0,'Beta',0);
end
%U(n-1)
if isempty(Pre_U)
    Pre_U  = struct('Alpha',0,'Beta',0);
end
%Estimated Back emf
if isempty(Est_E)
    Est_E  = struct('Alpha',0,'Beta',0);
end

if isempty(Error_I)
    Error_I = struct('Alpha',0,'Beta',0);
end

if isempty(Z)
    Z   = struct('Alpha',0,'Beta',0);
end

Pre_U.Alpha = U_Alpha;
Pre_U.Beta  = U_Beta;


%Estimated Current
Est_I.Alpha  = F * Est_I.Alpha + G*(Pre_U.Alpha - Z.Alpha);
Est_I.Beta   = F * Est_I.Beta  + G*(Pre_U.Beta    - Z.Beta);

%Error of Current
Error_I.Alpha = Est_I.Alpha - I_Alpha;
Error_I.Beta  = Est_I.Beta  - I_Beta;

%Sliding Mode 
if abs(Error_I.Alpha) > Error
  if Error_I.Alpha >= 0
     Z.Alpha = Kslide;
  else
     Z.Alpha = -Kslide; 
  end
else
  Z.Alpha = Kslide*(Error_I.Alpha/Error);
end

if abs(Error_I.Beta) > Error
  if Error_I.Beta >= 0
     Z.Beta = Kslide;
  else
     Z.Beta= -Kslide; 
  end
else
  Z.Beta = Kslide*(Error_I.Beta/Error);
end

%Estimated Back emf

Est_E.Alpha = Est_E.Alpha + Kslf* (Z.Alpha - Est_E.Alpha);
Est_E.Beta  = Est_E.Beta  + Kslf* (Z.Beta  - Est_E.Beta);

E_Alpha = Est_E.Alpha;
E_Beta  = Est_E.Beta;


Est_Ia=Est_I.Alpha;
Est_Ib=Est_I.Beta ;
